simulink model "SWC_InpMgmt_AFE"  (R2022b)
settings: configuration reference "DC_DC_Charger_Configuration" (kept outside this file)
values from neighbouring files (symbols this model uses):
  DC_VOLT_ADC_GAIN = 4095/3.3/2    (= 620.454545455)    [ConfigMe_AFE.m]    (also in SWC_InpMgmt_AFE.sldd = 620.454545454545
                
                    
     ; check_SWC_InpMgmt_AFE.sldd = 620.454545454545
                
                    
     )
  DC_VOLT_SNSR_GAIN = 3.3/1000    (= 0.0033)    [ConfigMe_AFE.m]    (also in SWC_InpMgmt_AFE.sldd = 0.0033
                
                    
               ; check_SWC_InpMgmt_AFE.sldd = 0.0033
                
                    
               )
  GRID_CURR_ADC_GAIN = 4096/3.3/2    (= 620.606060606)    [ConfigMe_AFE.m]    (also in SWC_InpMgmt_AFE.sldd = 620.60606060606
                
                    
      ; check_SWC_InpMgmt_AFE.sldd = 620.60606060606
                
                    
      )
  GRID_CURR_SNSR_GAIN = 3.3/50/1.414    (= 0.046676096181)    [ConfigMe_AFE.m]    (also in SWC_InpMgmt_AFE.sldd = 0.0466760961810466
                
                    
   ; check_SWC_InpMgmt_AFE.sldd = 0.0466760961810466
                
                    
   )
  GRID_VOLT_ADC_GAIN = 4095/3.3/2    (= 620.454545455)    [ConfigMe_AFE.m]    (also in SWC_InpMgmt_AFE.sldd = 620.4545455
                
                    
          ; check_SWC_InpMgmt_AFE.sldd = 620.4545455
                
                    
          )
  GRID_VOLT_SNSR_GAIN = 3.3/240/1.414    (= 0.00972418670438)    [ConfigMe_AFE.m]    (also in SWC_InpMgmt_AFE.sldd = 0.009724187
                
                    
          ; check_SWC_InpMgmt_AFE.sldd = 0.009724187
                
                    
          )
libraries: common_lib x12
settings Model: DataDictionary=SWC_InpMgmt_AFE.sldd  SimulationMode=accelerator  ExtModeTrigDuration=8  Creator=E0654638  LastModifiedBy=E0660158
settings ConfigSetRef: SourceName=DC_DC_Charger_Configuration

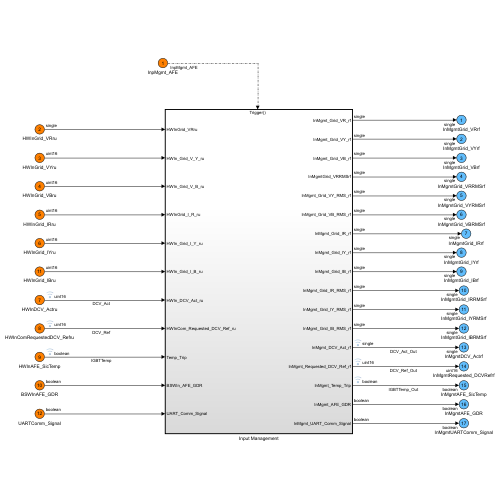
[thumbnail: Simulink's stored preview of the top-level diagram]
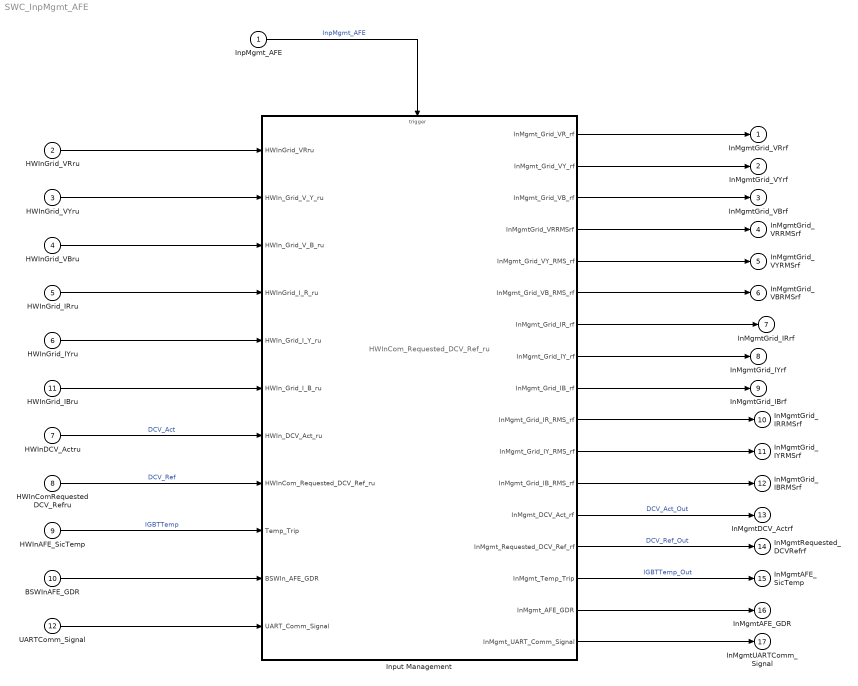
== system SWC_InpMgmt_AFE ==
  note: HWInCom_Requested_DCV_Ref_ru
  InpMgmt_AFE : Inport  Description=Inverter HVDC voltage  OutMin=0  OutMax=1000  PortDimensions=1  SampleTime=0.001  OutputFunctionCall=on
  HWInGrid_VRru : Inport  Port=2  OutDataTypeStr=single
  HWInGrid_VYru : Inport  Port=3  OutDataTypeStr=uint16
  HWInGrid_VBru : Inport  Port=4  OutDataTypeStr=uint16
  HWInGrid_IRru : Inport  Port=5  OutDataTypeStr=uint16
  HWInGrid_IYru : Inport  Port=6  OutDataTypeStr=uint16
  HWInDCV_Actru : Inport  Port=7  OutDataTypeStr=uint16
  HWInComRequestedDCV_Refru : Inport  Port=8  OutDataTypeStr=uint16
  HWInAFE_SicTemp : Inport  Port=9  OutDataTypeStr=boolean
  BSWInAFE_GDR : Inport  Port=10  OutDataTypeStr=boolean
  HWInGrid_IBru : Inport  Port=11  OutDataTypeStr=uint16
  UARTComm_Signal : Inport  Port=12  OutDataTypeStr=boolean
  Input Management : Subsystem
  InMgmtGrid_VRrf : Outport  OutDataTypeStr=single  VectorParamsAs1DForOutWhenUnconnected=off
  InMgmtGrid_VYrf : Outport  Port=2  OutDataTypeStr=single  VectorParamsAs1DForOutWhenUnconnected=off
  InMgmtGrid_VBrf : Outport  Port=3  OutDataTypeStr=single  VectorParamsAs1DForOutWhenUnconnected=off
  InMgmtGrid_VRRMSrf : Outport  Port=4  OutDataTypeStr=single  VectorParamsAs1DForOutWhenUnconnected=off
  InMgmtGrid_VYRMSrf : Outport  Port=5  OutDataTypeStr=single  VectorParamsAs1DForOutWhenUnconnected=off
  InMgmtGrid_VBRMSrf : Outport  Port=6  OutDataTypeStr=single  VectorParamsAs1DForOutWhenUnconnected=off
  InMgmtGrid_IRrf : Outport  Port=7  OutDataTypeStr=single  VectorParamsAs1DForOutWhenUnconnected=off
  InMgmtGrid_IYrf : Outport  Port=8  OutDataTypeStr=single  VectorParamsAs1DForOutWhenUnconnected=off
  InMgmtGrid_IBrf : Outport  Port=9  OutDataTypeStr=single  VectorParamsAs1DForOutWhenUnconnected=off
  InMgmtGrid_IRRMSrf : Outport  Port=10  OutDataTypeStr=single  VectorParamsAs1DForOutWhenUnconnected=off
  InMgmtGrid_IYRMSrf : Outport  Port=11  OutDataTypeStr=single  VectorParamsAs1DForOutWhenUnconnected=off
  InMgmtGrid_IBRMSrf : Outport  Port=12  OutDataTypeStr=single  VectorParamsAs1DForOutWhenUnconnected=off
  InMgmtDCV_Actrf : Outport  Port=13  OutDataTypeStr=single  VectorParamsAs1DForOutWhenUnconnected=off
  InMgmtRequested_DCVRefrf : Outport  Port=14  OutDataTypeStr=uint16  VectorParamsAs1DForOutWhenUnconnected=off
  InMgmtAFE_SicTemp : Outport  Port=15  OutDataTypeStr=boolean  VectorParamsAs1DForOutWhenUnconnected=off
  InMgmtAFE_GDR : Outport  Port=16  OutDataTypeStr=boolean  VectorParamsAs1DForOutWhenUnconnected=off
  InMgmtUARTComm_Signal : Outport  Port=17  OutDataTypeStr=boolean  VectorParamsAs1DForOutWhenUnconnected=off
  wires:
  InpMgmt_AFE/1 -> Input Management/Trigger  "InpMgmt_AFE"
  HWInDCV_Actru/1 -> Input Management/7(HWIn_DCV_Act_ru)  "DCV_Act"
  HWInComRequestedDCV_Refru/1 -> Input Management/8(HWInCom_Requested_DCV_Ref_ru)  "DCV_Ref"
  Input Management/14(InMgmt_Requested_DCV_Ref_rf) -> InMgmtRequested_DCVRefrf/1  "DCV_Ref_Out"
  Input Management/13(InMgmt_DCV_Act_rf) -> InMgmtDCV_Actrf/1  "DCV_Act_Out"
  Input Management/4(InMgmtGrid_VRRMSrf) -> InMgmtGrid_VRRMSrf/1
  HWInAFE_SicTemp/1 -> Input Management/9(Temp_Trip)  "IGBTTemp"
  BSWInAFE_GDR/1 -> Input Management/10(BSWIn_AFE_GDR)
  Input Management/16(InMgmt_AFE_GDR) -> InMgmtAFE_GDR/1
  Input Management/15(InMgmt_Temp_Trip) -> InMgmtAFE_SicTemp/1  "IGBTTemp_Out"
  HWInGrid_IBru/1 -> Input Management/6(HWIn_Grid_I_B_ru)
  HWInGrid_IYru/1 -> Input Management/5(HWIn_Grid_I_Y_ru)
  HWInGrid_IRru/1 -> Input Management/4(HWInGrid_I_R_ru)
  HWInGrid_VBru/1 -> Input Management/3(HWIn_Grid_V_B_ru)
  HWInGrid_VYru/1 -> Input Management/2(HWIn_Grid_V_Y_ru)
  HWInGrid_VRru/1 -> Input Management/1(HWInGrid_VRru)
  Input Management/12(InMgmt_Grid_IB_RMS_rf) -> InMgmtGrid_IBRMSrf/1
  Input Management/11(InMgmt_Grid_IY_RMS_rf) -> InMgmtGrid_IYRMSrf/1
  Input Management/10(InMgmt_Grid_IR_RMS_rf) -> InMgmtGrid_IRRMSrf/1
  Input Management/5(InMgmt_Grid_VY_RMS_rf) -> InMgmtGrid_VYRMSrf/1
  Input Management/6(InMgmt_Grid_VB_RMS_rf) -> InMgmtGrid_VBRMSrf/1
  UARTComm_Signal/1 -> Input Management/11(UART_Comm_Signal)
  Input Management/17(InMgmt_UART_Comm_Signal) -> InMgmtUARTComm_Signal/1
  Input Management/9(InMgmt_Grid_IB_rf) -> InMgmtGrid_IBrf/1
  Input Management/8(InMgmt_Grid_IY_rf) -> InMgmtGrid_IYrf/1
  Input Management/7(InMgmt_Grid_IR_rf) -> InMgmtGrid_IRrf/1
  Input Management/1(InMgmt_Grid_VR_rf) -> InMgmtGrid_VRrf/1
  Input Management/2(InMgmt_Grid_VY_rf) -> InMgmtGrid_VYrf/1
  Input Management/3(InMgmt_Grid_VB_rf) -> InMgmtGrid_VBrf/1

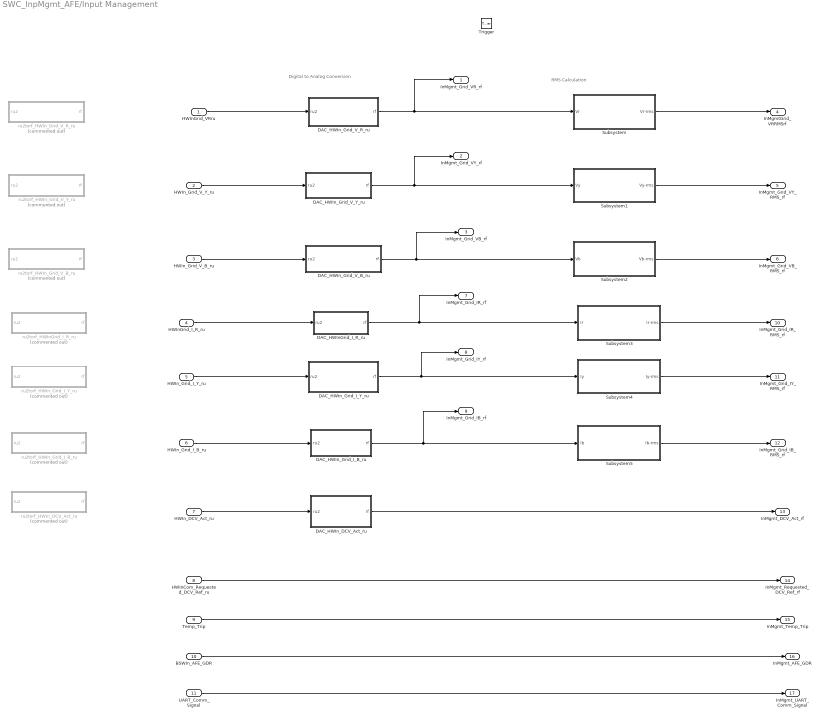
== system SWC_InpMgmt_AFE/Input Management ==
  note: RMS Calculation
  note: Digital to Analog Conversion
  HWInGrid_VRru : Inport
  HWIn_Grid_V_Y_ru : Inport  Port=2
  HWIn_Grid_V_B_ru : Inport  Port=3
  HWInGrid_I_R_ru : Inport  Port=4
  HWIn_Grid_I_Y_ru : Inport  Port=5
  HWIn_Grid_I_B_ru : Inport  Port=6
  HWIn_DCV_Act_ru : Inport  Port=7
  HWInCom_Requested_DCV_Ref_ru : Inport  Port=8
  Temp_Trip : Inport  Port=9
  BSWIn_AFE_GDR : Inport  Port=10
  UART_Comm_Signal : Inport  Port=11
  Trigger : TriggerPort  TriggerType=function-call  VariantControl=(inherit)  SampleTimeType=periodic  SampleTime=-1  PortDimensions=1
  DAC_HWInGrid_I_R_ru : Subsystem
  DAC_HWIn_DCV_Act_ru : Subsystem
  DAC_HWIn_Grid_I_B_ru : Subsystem
  DAC_HWIn_Grid_I_Y_ru : Subsystem
  DAC_HWIn_Grid_V_B_ru : Subsystem
  DAC_HWIn_Grid_V_R_ru : Subsystem
  DAC_HWIn_Grid_V_Y_ru : Subsystem
  Subsystem : Subsystem
  Subsystem1 : Subsystem
  Subsystem2 : Subsystem
  Subsystem3 : Subsystem
  Subsystem4 : Subsystem
  Subsystem5 : Subsystem
  ru2torf_HWInGrid_I_R_ru : Subsystem  Commented=on  mask{Offset_Value=2048, Gain_Value=GRID_CURR_SNSR_GAIN*GRID_CURR_ADC_GAIN}
      mask DialogControl ParameterGroupVar Prompt: Offset
      mask DialogControl ParameterGroupVar_copy Prompt: Gain
  ru2torf_HWIn_DCV_Act_ru : Subsystem  Commented=on  mask{Offset_Value=0, Gain_Value=DC_VOLT_ADC_GAIN*DC_VOLT_SNSR_GAIN}
      mask DialogControl ParameterGroupVar Prompt: Offset
      mask DialogControl ParameterGroupVar_copy Prompt: Gain
  ru2torf_HWIn_Grid_I_B_ru : Subsystem  Commented=on  mask{Offset_Value=2048, Gain_Value=GRID_CURR_SNSR_GAIN*GRID_CURR_ADC_GAIN}
      mask DialogControl ParameterGroupVar Prompt: Offset
      mask DialogControl ParameterGroupVar_copy Prompt: Gain
  ru2torf_HWIn_Grid_I_Y_ru : Subsystem  Commented=on  mask{Offset_Value=2048, Gain_Value=GRID_CURR_SNSR_GAIN*GRID_CURR_ADC_GAIN}
      mask DialogControl ParameterGroupVar Prompt: Offset
      mask DialogControl ParameterGroupVar_copy Prompt: Gain
  ru2torf_HWIn_Grid_V_B_ru : Subsystem  Commented=on  mask{Offset_Value=2048, Gain_Value=GRID_VOLT_SNSR_GAIN*GRID_VOLT_ADC_GAIN}
      mask DialogControl ParameterGroupVar Prompt: Offset
      mask DialogControl ParameterGroupVar_copy Prompt: Gain
  ru2torf_HWIn_Grid_V_R_ru : Subsystem  Commented=on  mask{Offset_Value=2048, Gain_Value=GRID_VOLT_SNSR_GAIN*GRID_VOLT_ADC_GAIN}
      mask DialogControl ParameterGroupVar Prompt: Offset
      mask DialogControl ParameterGroupVar_copy Prompt: Gain
  ru2torf_HWIn_Grid_V_Y_ru : Subsystem  Commented=on  mask{Offset_Value=2048, Gain_Value=GRID_VOLT_SNSR_GAIN*GRID_VOLT_ADC_GAIN}
      mask DialogControl ParameterGroupVar Prompt: Offset
      mask DialogControl ParameterGroupVar_copy Prompt: Gain
  InMgmt_Grid_VR_rf : Outport
  InMgmt_Grid_VY_rf : Outport  Port=2
  InMgmt_Grid_VB_rf : Outport  Port=3
  InMgmtGrid_VRRMSrf : Outport  Port=4
  InMgmt_Grid_VY_RMS_rf : Outport  Port=5
  InMgmt_Grid_VB_RMS_rf : Outport  Port=6
  InMgmt_Grid_IR_rf : Outport  Port=7
  InMgmt_Grid_IY_rf : Outport  Port=8
  InMgmt_Grid_IB_rf : Outport  Port=9
  InMgmt_Grid_IR_RMS_rf : Outport  Port=10
  InMgmt_Grid_IY_RMS_rf : Outport  Port=11
  InMgmt_Grid_IB_RMS_rf : Outport  Port=12
  InMgmt_DCV_Act_rf : Outport  Port=13
  InMgmt_Requested_DCV_Ref_rf : Outport  Port=14
  InMgmt_Temp_Trip : Outport  Port=15
  InMgmt_AFE_GDR : Outport  Port=16
  InMgmt_UART_Comm_Signal : Outport  Port=17
  wires:
  HWIn_Grid_I_Y_ru/1 -> DAC_HWIn_Grid_I_Y_ru/1(ru2)
  HWInGrid_I_R_ru/1 -> DAC_HWInGrid_I_R_ru/1(ru2)
  HWIn_Grid_I_B_ru/1 -> DAC_HWIn_Grid_I_B_ru/1(ru2)
  DAC_HWIn_Grid_V_R_ru/1(rf) -> Subsystem/1(Vr), InMgmt_Grid_VR_rf/1
  HWIn_DCV_Act_ru/1 -> DAC_HWIn_DCV_Act_ru/1(ru2)
  HWInGrid_VRru/1 -> DAC_HWIn_Grid_V_R_ru/1(ru2)
  HWIn_Grid_V_Y_ru/1 -> DAC_HWIn_Grid_V_Y_ru/1(ru2)
  HWIn_Grid_V_B_ru/1 -> DAC_HWIn_Grid_V_B_ru/1(ru2)
  Subsystem/1(Vr-rms) -> InMgmtGrid_VRRMSrf/1
  DAC_HWIn_Grid_V_Y_ru/1(rf) -> Subsystem1/1(Vy), InMgmt_Grid_VY_rf/1
  DAC_HWIn_Grid_V_B_ru/1(rf) -> Subsystem2/1(Vb), InMgmt_Grid_VB_rf/1
  Subsystem1/1(Vy-rms) -> InMgmt_Grid_VY_RMS_rf/1
  Subsystem2/1(Vb-rms) -> InMgmt_Grid_VB_RMS_rf/1
  DAC_HWIn_Grid_I_B_ru/1(rf) -> Subsystem5/1(Ib), InMgmt_Grid_IB_rf/1
  DAC_HWInGrid_I_R_ru/1(rf) -> Subsystem3/1(Ir), InMgmt_Grid_IR_rf/1
  DAC_HWIn_Grid_I_Y_ru/1(rf) -> Subsystem4/1(Iy), InMgmt_Grid_IY_rf/1
  Subsystem3/1(Ir-rms) -> InMgmt_Grid_IR_RMS_rf/1
  Subsystem4/1(Iy-rms) -> InMgmt_Grid_IY_RMS_rf/1
  Subsystem5/1(Ib-rms) -> InMgmt_Grid_IB_RMS_rf/1
  Temp_Trip/1 -> InMgmt_Temp_Trip/1
  BSWIn_AFE_GDR/1 -> InMgmt_AFE_GDR/1
  UART_Comm_Signal/1 -> InMgmt_UART_Comm_Signal/1
  HWInCom_Requested_DCV_Ref_ru/1 -> InMgmt_Requested_DCV_Ref_rf/1
  DAC_HWIn_DCV_Act_ru/1(rf) -> InMgmt_DCV_Act_rf/1

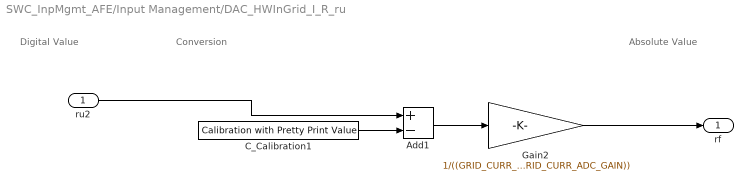
== system SWC_InpMgmt_AFE/Input Management/DAC_HWInGrid_I_R_ru ==
  note: Digital Value
  note: Conversion
  note: Absolute Value
  ru2 : Inport
  Add1 : Sum  Inputs=+-
  C_Calibration1 : common_lib/IO/Calibration with Pretty Print Value  CalValue=Offset_Value  scaling=None
  Gain2 : Gain  Gain=1/((GRID_CURR_SNSR_GAIN)*(GRID_CURR_ADC_GAIN))
  rf : Outport
  wires:
  C_Calibration1/1 -> Add1/2
  Gain2/1 -> rf/1
  ru2/1 -> Add1/1
  Add1/1 -> Gain2/1

== system SWC_InpMgmt_AFE/Input Management/DAC_HWIn_DCV_Act_ru ==
  note: Digital Value
  note: Absolute Value
  note: Conversion
  ru2 : Inport
  Gain2 : Gain  Gain=1/((DC_VOLT_SNSR_GAIN)*(DC_VOLT_ADC_GAIN))  OutDataTypeStr=single
  rf : Outport
  wires:
  Gain2/1 -> rf/1
  ru2/1 -> Gain2/1

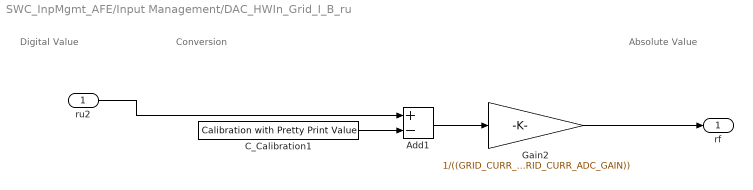
== system SWC_InpMgmt_AFE/Input Management/DAC_HWIn_Grid_I_B_ru ==
  note: Digital Value
  note: Conversion
  note: Absolute Value
  ru2 : Inport
  Add1 : Sum  Inputs=+-
  C_Calibration1 : common_lib/IO/Calibration with Pretty Print Value  CalValue=Offset_Value  scaling=None
  Gain2 : Gain  Gain=1/((GRID_CURR_SNSR_GAIN)*(GRID_CURR_ADC_GAIN))
  rf : Outport
  wires:
  C_Calibration1/1 -> Add1/2
  ru2/1 -> Add1/1
  Add1/1 -> Gain2/1
  Gain2/1 -> rf/1

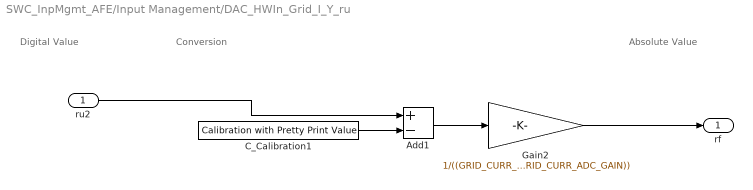
== system SWC_InpMgmt_AFE/Input Management/DAC_HWIn_Grid_I_Y_ru ==
  note: Absolute Value
  note: Digital Value
  note: Conversion
  ru2 : Inport
  Add1 : Sum  Inputs=+-
  C_Calibration1 : common_lib/IO/Calibration with Pretty Print Value  CalValue=Offset_Value  scaling=None
  Gain2 : Gain  Gain=1/((GRID_CURR_SNSR_GAIN)*(GRID_CURR_ADC_GAIN))
  rf : Outport
  wires:
  ru2/1 -> Add1/1
  C_Calibration1/1 -> Add1/2
  Gain2/1 -> rf/1
  Add1/1 -> Gain2/1

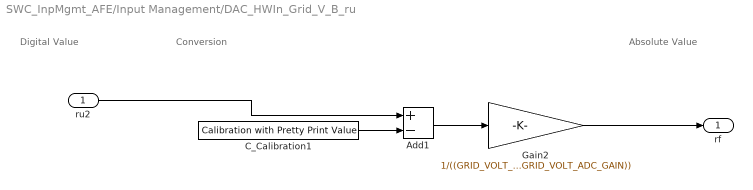
== system SWC_InpMgmt_AFE/Input Management/DAC_HWIn_Grid_V_B_ru ==
  note: Digital Value
  note: Conversion
  note: Absolute Value
  ru2 : Inport
  Add1 : Sum  Inputs=+-
  C_Calibration1 : common_lib/IO/Calibration with Pretty Print Value  CalValue=Offset_Value  scaling=None
  Gain2 : Gain  Gain=1/((GRID_VOLT_SNSR_GAIN)*(GRID_VOLT_ADC_GAIN))
  rf : Outport
  wires:
  C_Calibration1/1 -> Add1/2
  Gain2/1 -> rf/1
  Add1/1 -> Gain2/1
  ru2/1 -> Add1/1

== system SWC_InpMgmt_AFE/Input Management/DAC_HWIn_Grid_V_R_ru ==
  note: Conversion
  note: Absolute Value
  note: Digital Value
  ru2 : Inport
  Add1 : Sum  Inputs=+-
  C_Calibration1 : common_lib/IO/Calibration with Pretty Print Value  CalValue=Offset_Value  scaling=None
  Gain2 : Gain  Gain=1/((GRID_VOLT_SNSR_GAIN)*(GRID_VOLT_ADC_GAIN))
  rf : Outport
  wires:
  Gain2/1 -> rf/1
  C_Calibration1/1 -> Add1/2
  ru2/1 -> Add1/1
  Add1/1 -> Gain2/1

== system SWC_InpMgmt_AFE/Input Management/DAC_HWIn_Grid_V_Y_ru ==
  note: Conversion
  note: Digital Value
  note: Absolute Value
  ru2 : Inport
  Add1 : Sum  Inputs=+-
  C_Calibration1 : common_lib/IO/Calibration with Pretty Print Value  CalValue=Offset_Value  scaling=None
  Gain2 : Gain  Gain=1/((GRID_VOLT_SNSR_GAIN)*(GRID_VOLT_ADC_GAIN))
  rf : Outport
  wires:
  ru2/1 -> Add1/1
  Gain2/1 -> rf/1
  Add1/1 -> Gain2/1
  C_Calibration1/1 -> Add1/2

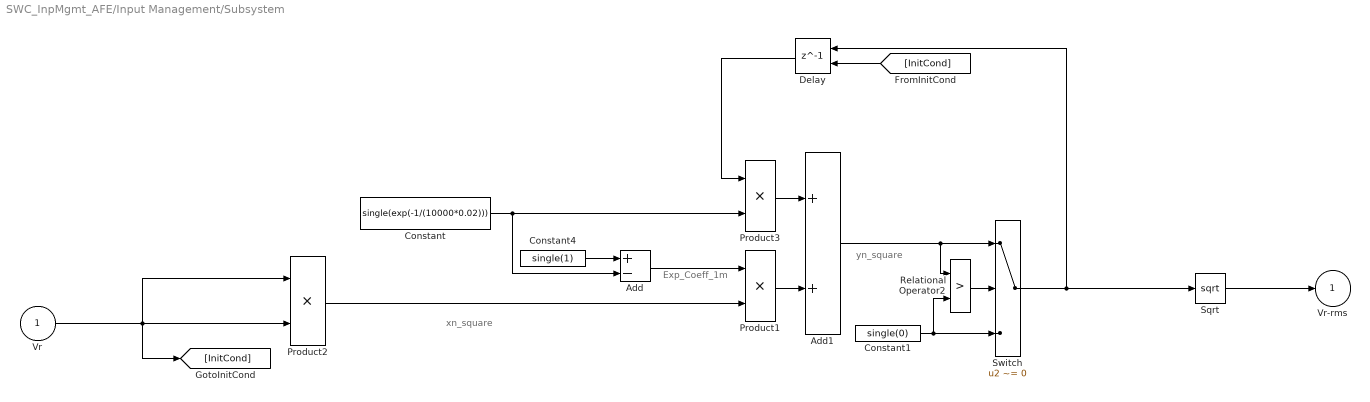
== system SWC_InpMgmt_AFE/Input Management/Subsystem ==
  note: Exp_Coeff_1m
  note: xn_square
  note: yn_square
  Vr : Inport
  Add : Sum  Inputs=+-
  Add1 : Sum
  Constant : Constant  Value=single(exp(-1/(10000*0.02)))  VectorParams1D=off
  Constant1 : Constant  Value=single(0)  SampleTime=-1
  Constant4 : Constant  Value=single(1)  SampleTime=-1
  Delay : Delay  DelayLength=1  InitialConditionSource=Input port
      settings: InputPortMap=u0,p4
  Product1 : Product
  Product2 : Product
  Product3 : Product
  Relational Operator2 : RelationalOperator  Operator=>  ZeroCross=off  RndMeth=Floor  InputSameDT=off
  Sqrt : Sqrt  SaturateOnIntegerOverflow=off
  Switch : Switch  Criteria=u2 ~= 0  Threshold=0.5  ZeroCross=off  SaturateOnIntegerOverflow=off  InputSameDT=off
  Vr-rms : Outport  VectorParamsAs1DForOutWhenUnconnected=off
  wires:
  Constant/1 -> Product3/2, Add/2
  Relational Operator2/1 -> Switch/2
  Constant4/1 -> Add/1
  Product3/1 -> Add1/1
  [InitCond] -> Delay/2
  Sqrt/1 -> Vr-rms/1
  Product1/1 -> Add1/2
  Constant1/1 -> Switch/3, Relational Operator2/2
  Switch/1 -> Delay/1, Sqrt/1
  Delay/1 -> Product3/1
  Add/1 -> Product1/1
  Add1/1 -> Relational Operator2/1, Switch/1
  Vr/1 -> Product2/1, [InitCond], Product2/2
  Product2/1 -> Product1/2

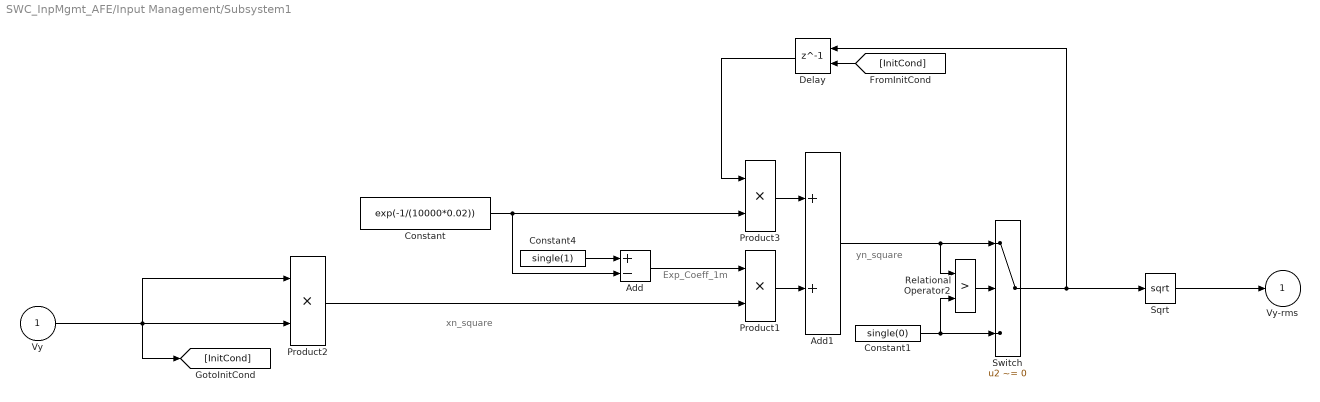
== system SWC_InpMgmt_AFE/Input Management/Subsystem1 ==
  note: yn_square
  note: xn_square
  note: Exp_Coeff_1m
  Vy : Inport
  Add : Sum  Inputs=+-
  Add1 : Sum
  Constant : Constant  Value=exp(-1/(10000*0.02))  VectorParams1D=off  OutDataTypeStr=single
  Constant1 : Constant  Value=single(0)  SampleTime=-1
  Constant4 : Constant  Value=single(1)  SampleTime=-1
  Delay : Delay  DelayLength=1  InitialConditionSource=Input port
      settings: InputPortMap=u0,p4
  Product1 : Product
  Product2 : Product
  Product3 : Product
  Relational Operator2 : RelationalOperator  Operator=>  ZeroCross=off  RndMeth=Floor  InputSameDT=off
  Sqrt : Sqrt  SaturateOnIntegerOverflow=off
  Switch : Switch  Criteria=u2 ~= 0  Threshold=0.5  ZeroCross=off  SaturateOnIntegerOverflow=off  InputSameDT=off
  Vy-rms : Outport  VectorParamsAs1DForOutWhenUnconnected=off
  wires:
  Product2/1 -> Product1/2
  Vy/1 -> Product2/2, [InitCond], Product2/1
  Add1/1 -> Switch/1, Relational Operator2/1
  Add/1 -> Product1/1
  Delay/1 -> Product3/1
  Switch/1 -> Sqrt/1, Delay/1
  Constant1/1 -> Switch/3, Relational Operator2/2
  Product1/1 -> Add1/2
  Sqrt/1 -> Vy-rms/1
  [InitCond] -> Delay/2
  Product3/1 -> Add1/1
  Constant4/1 -> Add/1
  Relational Operator2/1 -> Switch/2
  Constant/1 -> Add/2, Product3/2

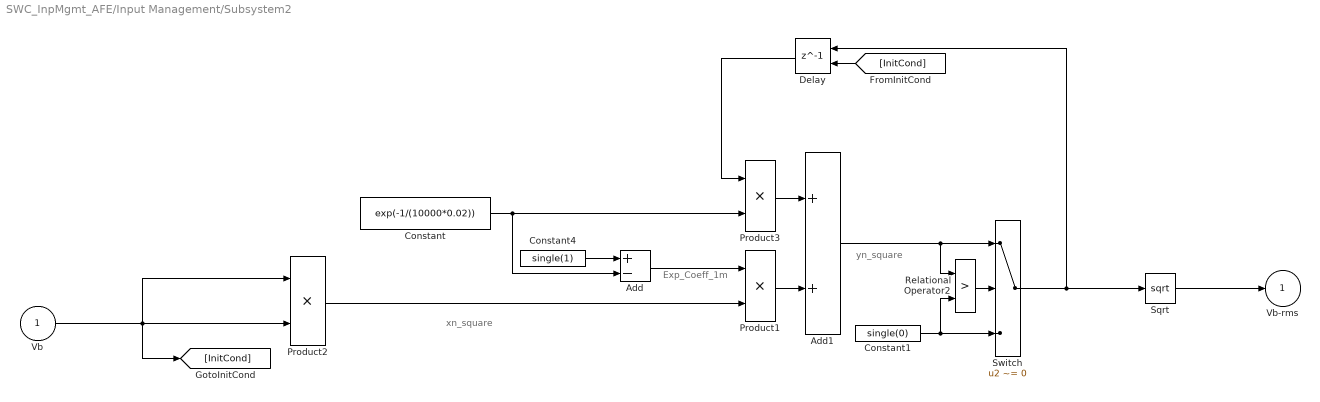
== system SWC_InpMgmt_AFE/Input Management/Subsystem2 ==
  note: Exp_Coeff_1m
  note: xn_square
  note: yn_square
  Vb : Inport
  Add : Sum  Inputs=+-
  Add1 : Sum
  Constant : Constant  Value=exp(-1/(10000*0.02))  VectorParams1D=off  OutDataTypeStr=single
  Constant1 : Constant  Value=single(0)  SampleTime=-1
  Constant4 : Constant  Value=single(1)  SampleTime=-1
  Delay : Delay  DelayLength=1  InitialConditionSource=Input port
      settings: InputPortMap=u0,p4
  Product1 : Product
  Product2 : Product
  Product3 : Product
  Relational Operator2 : RelationalOperator  Operator=>  ZeroCross=off  RndMeth=Floor  InputSameDT=off
  Sqrt : Sqrt  SaturateOnIntegerOverflow=off
  Switch : Switch  Criteria=u2 ~= 0  Threshold=0.5  ZeroCross=off  SaturateOnIntegerOverflow=off  InputSameDT=off
  Vb-rms : Outport  VectorParamsAs1DForOutWhenUnconnected=off
  wires:
  Constant/1 -> Product3/2, Add/2
  Relational Operator2/1 -> Switch/2
  Constant4/1 -> Add/1
  Product3/1 -> Add1/1
  [InitCond] -> Delay/2
  Sqrt/1 -> Vb-rms/1
  Product1/1 -> Add1/2
  Constant1/1 -> Relational Operator2/2, Switch/3
  Switch/1 -> Delay/1, Sqrt/1
  Delay/1 -> Product3/1
  Add/1 -> Product1/1
  Add1/1 -> Relational Operator2/1, Switch/1
  Vb/1 -> Product2/1, [InitCond], Product2/2
  Product2/1 -> Product1/2

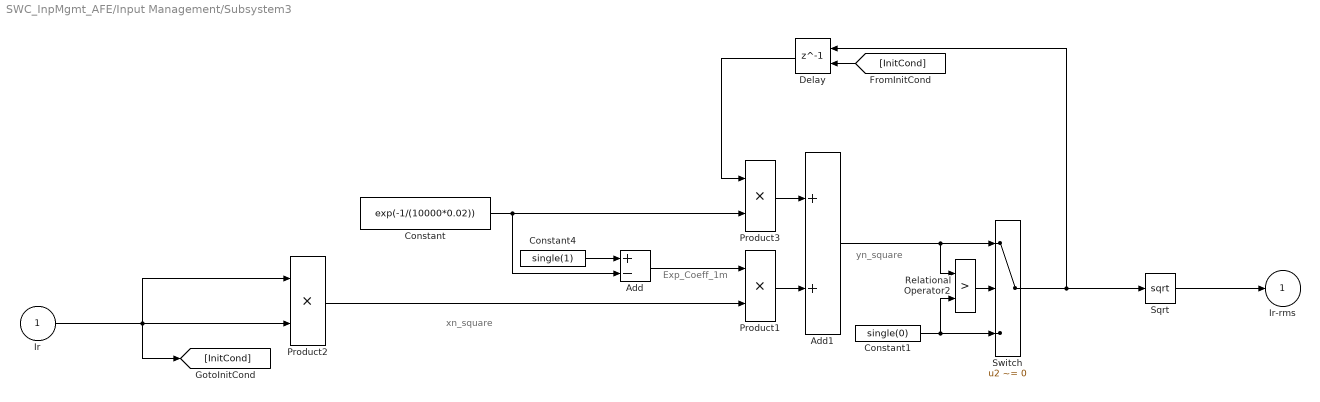
== system SWC_InpMgmt_AFE/Input Management/Subsystem3 ==
  note: yn_square
  note: xn_square
  note: Exp_Coeff_1m
  Ir : Inport
  Add : Sum  Inputs=+-
  Add1 : Sum
  Constant : Constant  Value=exp(-1/(10000*0.02))  VectorParams1D=off  OutDataTypeStr=single
  Constant1 : Constant  Value=single(0)  SampleTime=-1
  Constant4 : Constant  Value=single(1)  SampleTime=-1
  Delay : Delay  DelayLength=1  InitialConditionSource=Input port
      settings: InputPortMap=u0,p4
  Product1 : Product
  Product2 : Product
  Product3 : Product
  Relational Operator2 : RelationalOperator  Operator=>  ZeroCross=off  RndMeth=Floor  InputSameDT=off
  Sqrt : Sqrt  SaturateOnIntegerOverflow=off
  Switch : Switch  Criteria=u2 ~= 0  Threshold=0.5  ZeroCross=off  SaturateOnIntegerOverflow=off  InputSameDT=off
  Ir-rms : Outport  VectorParamsAs1DForOutWhenUnconnected=off
  wires:
  Product2/1 -> Product1/2
  Ir/1 -> Product2/2, [InitCond], Product2/1
  Add1/1 -> Switch/1, Relational Operator2/1
  Add/1 -> Product1/1
  Delay/1 -> Product3/1
  Switch/1 -> Sqrt/1, Delay/1
  Constant1/1 -> Switch/3, Relational Operator2/2
  Product1/1 -> Add1/2
  Sqrt/1 -> Ir-rms/1
  [InitCond] -> Delay/2
  Product3/1 -> Add1/1
  Constant4/1 -> Add/1
  Relational Operator2/1 -> Switch/2
  Constant/1 -> Add/2, Product3/2

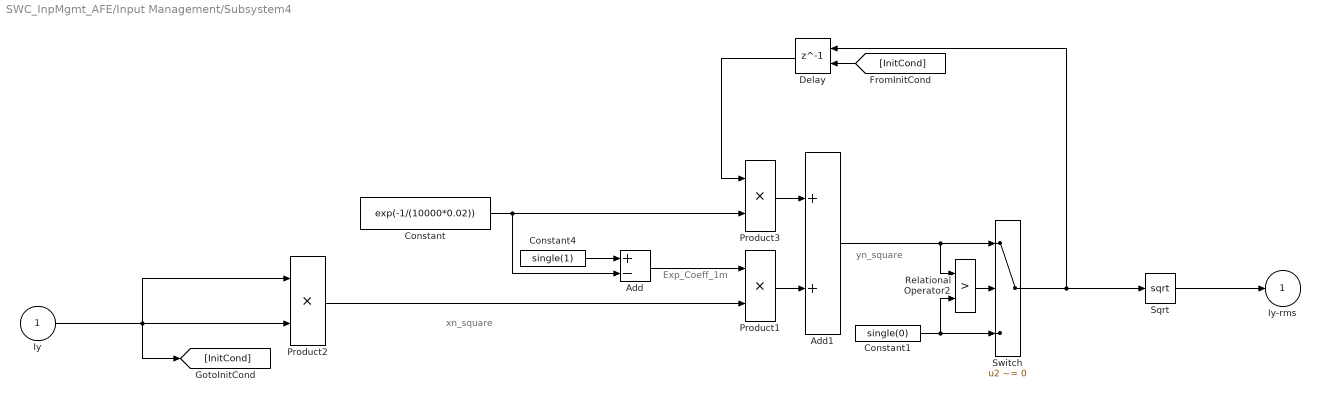
== system SWC_InpMgmt_AFE/Input Management/Subsystem4 ==
  note: Exp_Coeff_1m
  note: xn_square
  note: yn_square
  Iy : Inport
  Add : Sum  Inputs=+-
  Add1 : Sum
  Constant : Constant  Value=exp(-1/(10000*0.02))  VectorParams1D=off  OutDataTypeStr=single
  Constant1 : Constant  Value=single(0)  SampleTime=-1
  Constant4 : Constant  Value=single(1)  SampleTime=-1
  Delay : Delay  DelayLength=1  InitialConditionSource=Input port
      settings: InputPortMap=u0,p4
  Product1 : Product
  Product2 : Product
  Product3 : Product
  Relational Operator2 : RelationalOperator  Operator=>  ZeroCross=off  RndMeth=Floor  InputSameDT=off
  Sqrt : Sqrt  SaturateOnIntegerOverflow=off
  Switch : Switch  Criteria=u2 ~= 0  Threshold=0.5  ZeroCross=off  SaturateOnIntegerOverflow=off  InputSameDT=off
  Iy-rms : Outport  VectorParamsAs1DForOutWhenUnconnected=off
  wires:
  Constant/1 -> Product3/2, Add/2
  Relational Operator2/1 -> Switch/2
  Constant4/1 -> Add/1
  Product3/1 -> Add1/1
  [InitCond] -> Delay/2
  Sqrt/1 -> Iy-rms/1
  Product1/1 -> Add1/2
  Constant1/1 -> Relational Operator2/2, Switch/3
  Switch/1 -> Delay/1, Sqrt/1
  Delay/1 -> Product3/1
  Add/1 -> Product1/1
  Add1/1 -> Relational Operator2/1, Switch/1
  Iy/1 -> Product2/1, [InitCond], Product2/2
  Product2/1 -> Product1/2

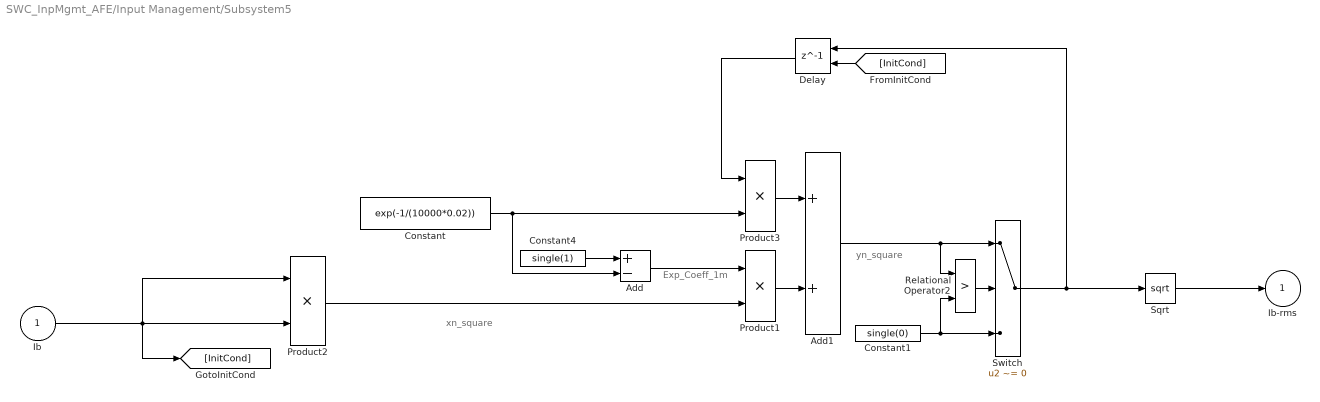
== system SWC_InpMgmt_AFE/Input Management/Subsystem5 ==
  note: yn_square
  note: xn_square
  note: Exp_Coeff_1m
  Ib : Inport
  Add : Sum  Inputs=+-
  Add1 : Sum
  Constant : Constant  Value=exp(-1/(10000*0.02))  VectorParams1D=off  OutDataTypeStr=single
  Constant1 : Constant  Value=single(0)  SampleTime=-1
  Constant4 : Constant  Value=single(1)  SampleTime=-1
  Delay : Delay  DelayLength=1  InitialConditionSource=Input port
      settings: InputPortMap=u0,p4
  Product1 : Product
  Product2 : Product
  Product3 : Product
  Relational Operator2 : RelationalOperator  Operator=>  ZeroCross=off  RndMeth=Floor  InputSameDT=off
  Sqrt : Sqrt  SaturateOnIntegerOverflow=off
  Switch : Switch  Criteria=u2 ~= 0  Threshold=0.5  ZeroCross=off  SaturateOnIntegerOverflow=off  InputSameDT=off
  Ib-rms : Outport  VectorParamsAs1DForOutWhenUnconnected=off
  wires:
  Product2/1 -> Product1/2
  Ib/1 -> Product2/1, Product2/2, [InitCond]
  Add1/1 -> Switch/1, Relational Operator2/1
  Add/1 -> Product1/1
  Delay/1 -> Product3/1
  Switch/1 -> Sqrt/1, Delay/1
  Constant1/1 -> Switch/3, Relational Operator2/2
  Product1/1 -> Add1/2
  Sqrt/1 -> Ib-rms/1
  [InitCond] -> Delay/2
  Product3/1 -> Add1/1
  Constant4/1 -> Add/1
  Relational Operator2/1 -> Switch/2
  Constant/1 -> Add/2, Product3/2

== system SWC_InpMgmt_AFE/Input Management/ru2torf_HWInGrid_I_R_ru ==
  note: Conversion
  note: Absolute Value
  note: Digital Value
  ru2 : Inport
  Add1 : Sum  Inputs=+-
  C_Calibration1 : common_lib/IO/Calibration with Pretty Print Value  CalValue=Offset_Value  scaling=None
  Gain2 : Gain  Gain=1/((GRID_CURR_SNSR_GAIN)*(GRID_CURR_ADC_GAIN))  OutDataTypeStr=uint16
  rf : Outport
  wires:
  Gain2/1 -> rf/1
  ru2/1 -> Add1/1
  C_Calibration1/1 -> Add1/2
  Add1/1 -> Gain2/1

== system SWC_InpMgmt_AFE/Input Management/ru2torf_HWIn_DCV_Act_ru ==
  note: Digital Value
  note: Absolute Value
  note: Conversion
  ru2 : Inport
  Gain2 : Gain  Gain=1/((DC_VOLT_SNSR_GAIN)*(DC_VOLT_ADC_GAIN))  OutDataTypeStr=uint16
  rf : Outport
  wires:
  ru2/1 -> Gain2/1
  Gain2/1 -> rf/1

== system SWC_InpMgmt_AFE/Input Management/ru2torf_HWIn_Grid_I_B_ru ==
  note: Conversion
  note: Absolute Value
  note: Digital Value
  ru2 : Inport
  Add1 : Sum  Inputs=+-
  C_Calibration1 : common_lib/IO/Calibration with Pretty Print Value  CalValue=Offset_Value  scaling=None
  Gain2 : Gain  Gain=1/((GRID_CURR_SNSR_GAIN)*(GRID_CURR_ADC_GAIN))  OutDataTypeStr=uint16
  rf : Outport
  wires:
  Gain2/1 -> rf/1
  ru2/1 -> Add1/1
  C_Calibration1/1 -> Add1/2
  Add1/1 -> Gain2/1

== system SWC_InpMgmt_AFE/Input Management/ru2torf_HWIn_Grid_I_Y_ru ==
  note: Digital Value
  note: Absolute Value
  note: Conversion
  ru2 : Inport
  Add1 : Sum  Inputs=+-
  C_Calibration1 : common_lib/IO/Calibration with Pretty Print Value  CalValue=Offset_Value  scaling=None
  Gain2 : Gain  Gain=1/((GRID_CURR_SNSR_GAIN)*(GRID_CURR_ADC_GAIN))  OutDataTypeStr=uint16
  rf : Outport
  wires:
  Add1/1 -> Gain2/1
  C_Calibration1/1 -> Add1/2
  ru2/1 -> Add1/1
  Gain2/1 -> rf/1

== system SWC_InpMgmt_AFE/Input Management/ru2torf_HWIn_Grid_V_B_ru ==
  note: Digital Value
  note: Absolute Value
  note: Conversion
  ru2 : Inport
  Add1 : Sum  Inputs=+-
  C_Calibration1 : common_lib/IO/Calibration with Pretty Print Value  CalValue=Offset_Value  scaling=None
  Gain2 : Gain  Gain=1/((GRID_VOLT_SNSR_GAIN)*(GRID_VOLT_ADC_GAIN))  OutDataTypeStr=uint16
  rf : Outport
  wires:
  Add1/1 -> Gain2/1
  C_Calibration1/1 -> Add1/2
  ru2/1 -> Add1/1
  Gain2/1 -> rf/1

== system SWC_InpMgmt_AFE/Input Management/ru2torf_HWIn_Grid_V_R_ru ==
  note: Digital Value
  note: Absolute Value
  note: Conversion
  ru2 : Inport
  Add1 : Sum  Inputs=+-
  C_Calibration1 : common_lib/IO/Calibration with Pretty Print Value  CalValue=Offset_Value  scaling=None
  Gain2 : Gain  Gain=1/((GRID_VOLT_SNSR_GAIN)*(GRID_VOLT_ADC_GAIN))  OutDataTypeStr=uint16
  rf : Outport
  wires:
  Add1/1 -> Gain2/1
  C_Calibration1/1 -> Add1/2
  ru2/1 -> Add1/1
  Gain2/1 -> rf/1

== system SWC_InpMgmt_AFE/Input Management/ru2torf_HWIn_Grid_V_Y_ru ==
  note: Conversion
  note: Absolute Value
  note: Digital Value
  ru2 : Inport
  Add1 : Sum  Inputs=+-
  C_Calibration1 : common_lib/IO/Calibration with Pretty Print Value  CalValue=Offset_Value  scaling=None
  Gain2 : Gain  Gain=1/((GRID_VOLT_SNSR_GAIN)*(GRID_VOLT_ADC_GAIN))  OutDataTypeStr=uint16
  rf : Outport
  wires:
  Gain2/1 -> rf/1
  ru2/1 -> Add1/1
  C_Calibration1/1 -> Add1/2
  Add1/1 -> Gain2/1
